simulink model "Task1"  (R2019b)
settings: Solver=FixedStepAuto  StartTime=0.0  StopTime=10.0  FixedStep=1e-4  RelTol=1e-3
settings Model: DataTypeOverride=Double  MinMaxOverflowLogging=ForceOff  Creator=sinow  LastModifiedBy=sinow

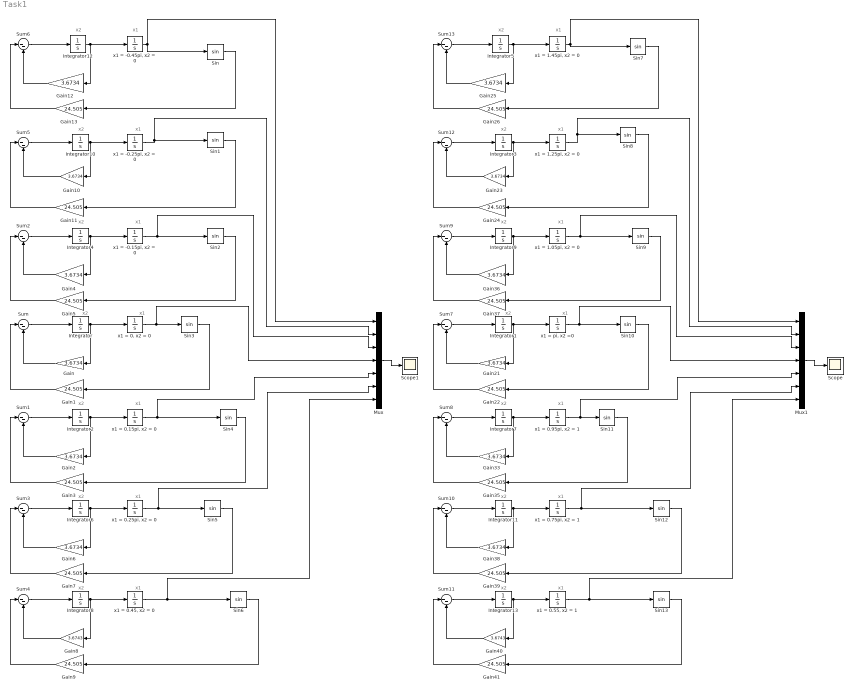
== system Task1 ==
  note: x1
  note: x2
  note: x2
  note: x1
  note: x2
  note: x1
  note: x2
  note: x1
  note: x2
  note: x1
  note: x2
  note: x1
  note: x2
  note: x1
  note: x1
  note: x2
  note: x2
  note: x1
  note: x2
  note: x1
  note: x2
  note: x1
  note: x1
  note: x1
  note: x2
  note: x2
  note: x1
  note: x2
  Gain{,2,4,6,10,12,21,23,25,33,36,38} (12 alike) : Gain  Gain=3.6734
  Gain{1,3,5,7,9,11,13,22,24,26,35,37,39,41} (14 alike) : Gain  Gain=24.505
  Gain40 : Gain  Gain=3.6743
  Gain8 : Gain  Gain=3.6743
  Integrator{,1..13} (14 alike) : Integrator
  Mux : Mux  Inputs=7
  Mux1 : Mux  Inputs=7
  Scope : Scope
  Scope1 : Scope
  Sin{,1..13} (14 alike) : Trigonometry
  Sum{,1..13} (14 alike) : Sum  Inputs=|--
  "x1 = -0.15pi, x2 = 0" : Integrator  InitialCondition=-0.15*pi
  "x1 = -0.25pi, x2 = 0" : Integrator  InitialCondition=-0.25*pi
  "x1 = -0.45pi, x2 = 0" : Integrator  InitialCondition=-0.45*pi
  "x1 = 0, x2 = 0" : Integrator
  "x1 = 0.15pi, x2 = 0" : Integrator  InitialCondition=0.15*pi
  "x1 = 0.25pi, x2 = 0" : Integrator  InitialCondition=0.25*pi
  "x1 = 0.45, x2 = 0" : Integrator  InitialCondition=0.45*pi
  "x1 = 0.55, x2 = 1" : Integrator  InitialCondition=0.55*pi
  "x1 = 0.75pi, x2 = 1" : Integrator  InitialCondition=0.75*pi
  "x1 = 0.95pi, x2 = 1" : Integrator  InitialCondition=0.95*pi
  "x1 = 1.05pi, x2 = 0" : Integrator  InitialCondition=1.05*pi
  "x1 = 1.25pi, x2 = 0" : Integrator  InitialCondition=1.25*pi
  "x1 = 1.45pi, x2 = 0" : Integrator  InitialCondition=1.45*pi
  "x1 = pi, x2 =0" : Integrator  InitialCondition=pi
  wires:
  Gain1/1 -> Sum/1
  Gain/1 -> Sum/2
  Sum/1 -> Integrator/1
  Integrator/1 -> Gain/1, "x1 = 0, x2 = 0"/1
  Sin3/1 -> Gain1/1
  Mux/1 -> Scope1/1
  Sin4/1 -> Gain3/1
  Integrator2/1 -> Gain2/1, "x1 = 0.15pi, x2 = 0"/1
  Gain3/1 -> Sum1/1
  Gain2/1 -> Sum1/2
  Sum1/1 -> Integrator2/1
  Gain4/1 -> Sum2/2
  Sum2/1 -> Integrator4/1
  Gain5/1 -> Sum2/1
  Sin2/1 -> Gain5/1
  Integrator4/1 -> Gain4/1, "x1 = -0.15pi, x2 = 0"/1
  Gain6/1 -> Sum3/2
  Sum3/1 -> Integrator6/1
  Gain7/1 -> Sum3/1
  Sin5/1 -> Gain7/1
  Integrator6/1 -> Gain6/1, "x1 = 0.25pi, x2 = 0"/1
  Gain8/1 -> Sum4/2
  Sum4/1 -> Integrator8/1
  Gain9/1 -> Sum4/1
  Integrator8/1 -> Gain8/1, "x1 = 0.45, x2 = 0"/1
  Gain10/1 -> Sum5/2
  Sum5/1 -> Integrator10/1
  Gain11/1 -> Sum5/1
  Sin1/1 -> Gain11/1
  Integrator10/1 -> Gain10/1, "x1 = -0.25pi, x2 = 0"/1
  Gain12/1 -> Sum6/2
  Sum6/1 -> Integrator12/1
  Gain13/1 -> Sum6/1
  Sin/1 -> Gain13/1
  Integrator12/1 -> Gain12/1, "x1 = -0.45pi, x2 = 0"/1
  Sin6/1 -> Gain9/1
  "x1 = -0.25pi, x2 = 0"/1 -> Sin1/1, Mux/2
  "x1 = -0.15pi, x2 = 0"/1 -> Sin2/1, Mux/3
  "x1 = 0, x2 = 0"/1 -> Sin3/1, Mux/4
  "x1 = 0.15pi, x2 = 0"/1 -> Sin4/1, Mux/5
  "x1 = 0.25pi, x2 = 0"/1 -> Sin5/1, Mux/6
  "x1 = 0.45, x2 = 0"/1 -> Sin6/1, Mux/7
  "x1 = -0.45pi, x2 = 0"/1 -> Sin/1, Mux/1
  Integrator13/1 -> Gain40/1, "x1 = 0.55, x2 = 1"/1
  Sin8/1 -> Gain24/1
  Integrator3/1 -> Gain23/1, "x1 = 1.25pi, x2 = 0"/1
  Gain36/1 -> Sum9/2
  "x1 = 1.45pi, x2 = 0"/1 -> Sin7/1, Mux1/1
  Sin12/1 -> Gain39/1
  Gain37/1 -> Sum9/1
  "x1 = 0.55, x2 = 1"/1 -> Sin13/1, Mux1/7
  Gain23/1 -> Sum12/2
  Gain41/1 -> Sum11/1
  Integrator5/1 -> Gain25/1, "x1 = 1.45pi, x2 = 0"/1
  Gain25/1 -> Sum13/2
  "x1 = pi, x2 =0"/1 -> Sin10/1, Mux1/4
  "x1 = 0.95pi, x2 = 1"/1 -> Sin11/1, Mux1/5
  Gain26/1 -> Sum13/1
  Sum12/1 -> Integrator3/1
  Sin9/1 -> Gain37/1
  Gain40/1 -> Sum11/2
  "x1 = 1.05pi, x2 = 0"/1 -> Sin9/1, Mux1/3
  Gain24/1 -> Sum12/1
  Sin13/1 -> Gain41/1
  Sum7/1 -> Integrator1/1
  Integrator11/1 -> Gain38/1, "x1 = 0.75pi, x2 = 1"/1
  Sum11/1 -> Integrator13/1
  Sin7/1 -> Gain26/1
  Gain39/1 -> Sum10/1
  Gain21/1 -> Sum7/2
  Integrator9/1 -> Gain36/1, "x1 = 1.05pi, x2 = 0"/1
  Sum13/1 -> Integrator5/1
  Sum8/1 -> Integrator7/1
  Gain33/1 -> Sum8/2
  "x1 = 0.75pi, x2 = 1"/1 -> Sin12/1, Mux1/6
  Integrator1/1 -> Gain21/1, "x1 = pi, x2 =0"/1
  Mux1/1 -> Scope/1
  Sin11/1 -> Gain35/1
  Integrator7/1 -> Gain33/1, "x1 = 0.95pi, x2 = 1"/1
  "x1 = 1.25pi, x2 = 0"/1 -> Sin8/1, Mux1/2
  Gain35/1 -> Sum8/1
  Gain38/1 -> Sum10/2
  Sum9/1 -> Integrator9/1
  Sin10/1 -> Gain22/1
  Gain22/1 -> Sum7/1
  Sum10/1 -> Integrator11/1
